simulink model "ssbdemo"  (Simulink 4.00)
settings: Solver=FixedStepDiscrete  SolverMode=SingleTasking  StartTime=0.0  StopTime=99999999  RelTol=1e-3  AbsTol=1e-6
libraries: dspsrcs3 x2, dspxfrm3 x1, dspsnks3 x1
settings Model: CovMetricSettings=d  Creator=don  LastModifiedBy=ashah  SaveTime=off  SaveOutput=off  LimitDataPoints=off  IntegerOverflowMsg=none  RTWOptions=-aRollThreshold=2  ExtModeTrigMode=oneshot  ExtModeArmWhenConnect=off  BlockReductionOpt=off

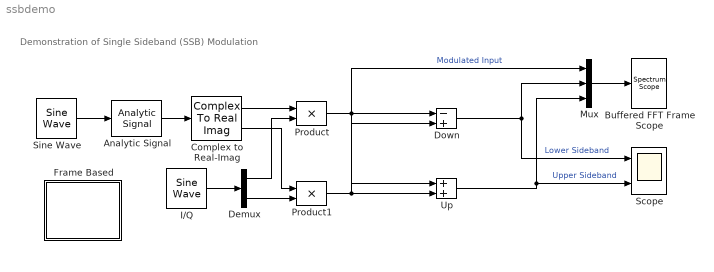
== system ssbdemo ==
  note: Demonstration of
      | Single Sideband (SSB)
      | Modulation
  Analytic Signal : dspxfrm3/Analytic Signal  N=100
  Buffered FFT Frame Scope : dspsnks3/Spectrum Scope  ScopeProperties=off  Domain=Frequency  HorizSpan=1  UseBuffer=on  BufferSize=128  Overlap=64  inpFftLenInherit=off  FFTlength=128  numAvg=1  DisplayProperties=off  AxisGrid=on  Memory=off  FrameNumber=off  AxisLegend=on  AxisZoom=off  OpenScopeAtSimStart=on  OpenScopeImmediately=off  FigPos=[399 256 382 346]  AxisProperties=on  XUnits=Hertz  XRange=[0...Fs/2]  InheritXIncr=on  XIncr=1  XLabel=Samples  YUnits=dB  YLabel=Magnitude, dB  LineProperties=off  LineColors=|[1 0 1]|[0 0 1]
      settings: YMin=-124.156289978703  YMax=13.9194893778784
  Complex to Real-Imag : ComplexToRealImag  Output=RealAndImag
  Demux : Demux  Outputs=2  BusSelectionMode=off
  Down : Sum  Inputs=-+  SaturateOnIntegerOverflow=on
  Frame Based : Subsystem
      settings: OpenFcn=ssbdemof;  RTWFcnNameOpts=Auto  RTWFileNameOpts=Auto
      mask Display: disp('Frame-based\nVersion')
  I/Q : dspsrcs3/Sine Wave  Amplitude=1  Frequency=2  Phase=[0 pi/2]  SampleMode=Discrete  OutComplex=Real  CompMethod=Trigonometric Fcn  TableSize=Speed  SampleTime=0.1  SamplesPerFrame=1  ResetState=Restart at time zero
  Mux : Mux  Inputs=3  BusCreatorMode=off
  Product : Product  Inputs=2  Multiplication=Element-wise(.*)  SaturateOnIntegerOverflow=on
  Product1 : Product  Inputs=2  Multiplication=Element-wise(.*)  SaturateOnIntegerOverflow=on
  Scope : Scope  NumInputPorts=2
      settings: TimeRange=3  YMin=-1.2~-1.2  YMax=1.2~1.2  SaveToWorkspace=off  SaveName=ScopeData  DataFormat=Array  LimitDataPoints=on  MaxDataPoints=5000
  Sine Wave : dspsrcs3/Sine Wave  Amplitude=1  Frequency=0.5  Phase=0  SampleMode=Discrete  OutComplex=Real  CompMethod=Trigonometric Fcn  TableSize=Speed  SampleTime=0.1  SamplesPerFrame=1  ResetState=Restart at time zero
  Up : Sum  Inputs=++  SaturateOnIntegerOverflow=on
  wires:
  Sine Wave/1 -> Analytic Signal/1
  Analytic Signal/1 -> Complex to Real-Imag/1
  Product/1 -> Down/1, Up/1, Mux/1  "Modulated Input"
  Product1/1 -> Up/2, Down/2
  Complex to Real-Imag/2 -> Product1/1
  Demux/2 -> Product1/2
  Complex to Real-Imag/1 -> Product/1
  Demux/1 -> Product/2
  Down/1 -> Scope/1, Mux/2  "Lower Sideband"
  Up/1 -> Mux/3, Scope/2  "Upper Sideband"
  I/Q/1 -> Demux/1
  Mux/1 -> Buffered FFT Frame Scope/1

== system ssbdemo/Frame Based ==
